simulink model "Trim"  (R2022b)
settings: Solver=ode4  StartTime=0.0  StopTime=30  FixedStep=0.01  RelTol=1e-3
undefined symbols (not defined in the file): Data, IC, Sim, v0_BE_B
libraries: simulink_extras x2, sharedutil x2
settings Model: PauseTimes=399.98  PacingRate=1000  Creator=Thoma  LastModifiedBy=muel_td
settings DataIOCC: ExternalInput=getinputstruct(report2)  InitialState=getstatestruct(report2)
settings OptimizationCC: ReuseModelBlockBuffer=on
settings DebuggingCC: AlgebraicLoopMsg=none  InitInArrayFormatMsg=none
settings RTWCC: GPUComputeCapability=5.0

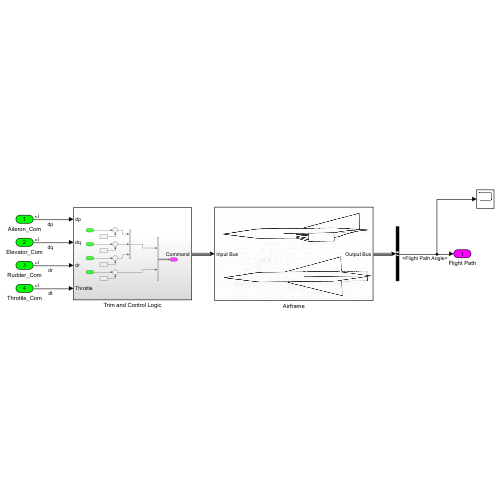
[thumbnail: Simulink's stored preview of the top-level diagram]
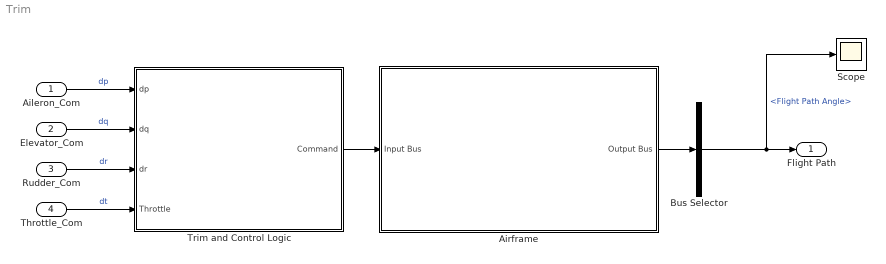
== system Trim ==
  Aileron_Com : Inport  OutDataTypeStr=double
  Elevator_Com : Inport  Port=2  OutDataTypeStr=double
  Rudder_Com : Inport  Port=3  OutDataTypeStr=double
  Throttle_Com : Inport  Port=4
  Airframe : Subsystem
      mask Display: image('GHAME.png'); % Use "Edit Image" on toolstrip to change.
  Bus Selector : BusSelector  OutputSignals=Flight Path Angle
  Scope : Scope
  Trim and Control Logic : Subsystem
  Flight Path : Outport
  wires:
  Airframe/1(Output Bus) -> Bus Selector/1
  Bus Selector/1 -> Scope/1, Flight Path/1  "<Flight Path Angle>"
  Aileron_Com/1 -> Trim and Control Logic/1(dp)  "dp"
  Elevator_Com/1 -> Trim and Control Logic/2(dq)  "dq"
  Rudder_Com/1 -> Trim and Control Logic/3(dr)  "dr"
  Throttle_Com/1 -> Trim and Control Logic/4(Throttle)  "dt"
  Trim and Control Logic/1(Command) -> Airframe/1(Input Bus)

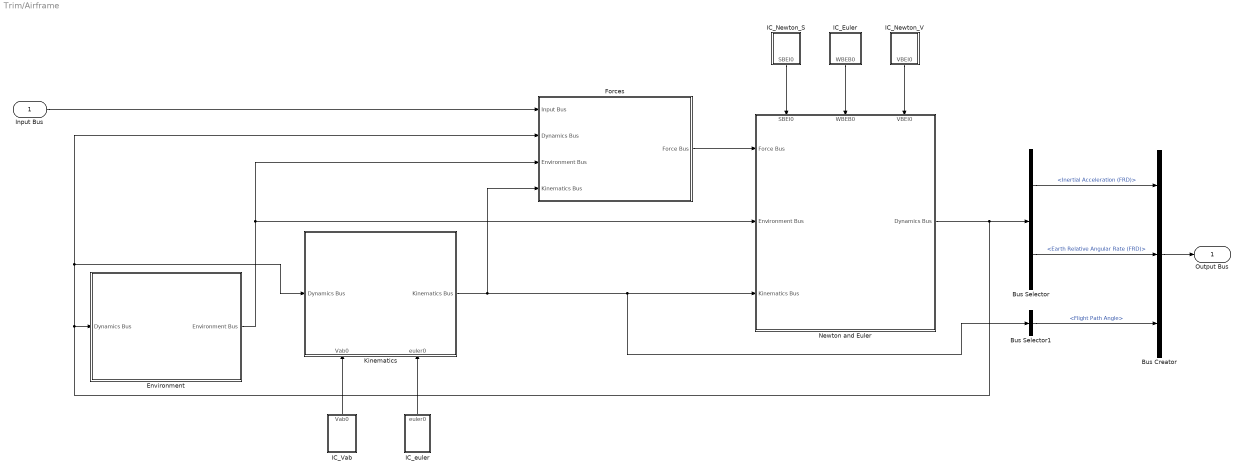
== system Trim/Airframe ==
  Input Bus : Inport
  Bus Creator : BusCreator  Inputs=3
  Bus Selector : BusSelector  OutputSignals=Inertial Acceleration (FRD),Earth Relative Angular Rate (FRD)
  Bus Selector1 : BusSelector  OutputSignals=Flight Path Angle
  Environment : Subsystem
  Forces : Subsystem
  IC_Euler : Subsystem
  IC_Newton_S : Subsystem
  IC_Newton_V : Subsystem
  IC_Vab : Subsystem
  IC_euler : Subsystem
  Kinematics : Subsystem
      settings: PortSchema="{\"entries\":[{\"content\":{\"sides\":[{\"content\":{\"connectorIds\":[\"In1\"]},\"type\":\"ConnectorPlacement.EquallySpacedRectSide\",\"uuid\":\"165cd628-1618-4ee0-958f-c15c2fb528e8\"},{\"content\":{\"connectorIds\":[\"Out1\"],\"side\":\"RIGHT\"},\"type\":\"ConnectorPlacement.EquallySpacedRectSide\",\"uuid\":\"946488ef-ac28-4d5b-ba51-e112409765b1\"},{\"content\":{\"connectorIds\":[],\"side\":\"TOP\"},\"type\":\"ConnectorPlacement.EquallySpacedRectSide\",\"uuid\":\"119c1b56-3e48-4508-9afd-e07e28cbf837\"},{\"content\":{\"connectorIds\":[\"In2\",\"In3\"],\"side\":\"BOTTOM\"},\"type\":\"ConnectorPlacement.EquallySpacedRectSide\",\"uuid\":\"d60bed97-cd35-4219-85e4-6b5accaebd4d\"}]},\"type\":\"ConnectorPlacement.EquallySpacedConnector\",\"uuid\":\"f554c72c-6bea-4d8c-bbaa-1d03e69e35ab\"}],\"packageUris\":[\"http://schema.mathworks.com/mf0/Connector/R2020b\"],\"version\":\"1.0\"}"
  Newton and Euler : Subsystem
      settings: PortSchema="{\"entries\":[{\"content\":{\"sides\":[{\"content\":{\"connectorIds\":[\"In1\",\"In2\",\"In3\"]},\"type\":\"ConnectorPlacement.EquallySpacedRectSide\",\"uuid\":\"2ee03a1f-357d-4786-8b32-c5c02601a636\"},{\"content\":{\"connectorIds\":[\"Out1\"],\"side\":\"RIGHT\"},\"type\":\"ConnectorPlacement.EquallySpacedRectSide\",\"uuid\":\"c5e575c4-9295-4acb-b0b8-b029d28de022\"},{\"content\":{\"connectorIds\":[\"In4\",\"In5\",\"In6\"],\"side\":\"TOP\"},\"type\":\"ConnectorPlacement.EquallySpacedRectSide\",\"uuid\":\"0c94ab65-bccb-43d1-9b54-9d35a0cc0e07\"}]},\"type\":\"ConnectorPlacement.EquallySpacedConnector\",\"uuid\":\"e611a102-f7b3-4598-9b4e-dc828ce04541\"}],\"packageUris\":[\"http://schema.mathworks.com/mf0/Connector/R2020b\"],\"version\":\"1.0\"}"
  Output Bus : Outport
  wires:
  Newton and Euler/1(Dynamics Bus) -> Environment/1(Dynamics Bus), Forces/2(Dynamics Bus), Kinematics/1(Dynamics Bus), Bus Selector/1
  IC_Newton_V/1(VBEI0) -> Newton and Euler/6(VBEI0)
  IC_Vab/1(Vab0) -> Kinematics/2(Vab0)
  IC_Euler/1(WBEB0) -> Newton and Euler/5(WBEB0)
  IC_Newton_S/1(SBEI0) -> Newton and Euler/4(SBEI0)
  Kinematics/1(Kinematics Bus) -> Forces/4(Kinematics Bus), Newton and Euler/3(Kinematics Bus), Bus Selector1/1
  IC_euler/1(euler0) -> Kinematics/3(euler0)
  Environment/1(Environment Bus) -> Forces/3(Environment Bus), Newton and Euler/2(Environment Bus)
  Forces/1(Force Bus) -> Newton and Euler/1(Force Bus)
  Input Bus/1 -> Forces/1(Input Bus)
  Bus Creator/1 -> Output Bus/1
  Bus Selector1/1 -> Bus Creator/3  "<Flight Path Angle>"
  Bus Selector/2 -> Bus Creator/2  "<Earth Relative Angular Rate (FRD)>"
  Bus Selector/1 -> Bus Creator/1  "<Inertial Acceleration (FRD)>"

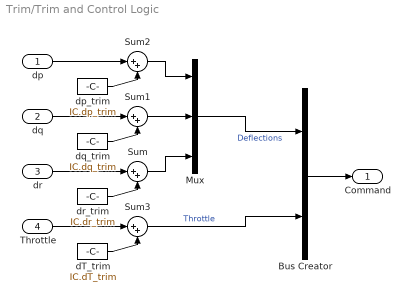
== system Trim/Trim and Control Logic ==
  dp : Inport
  dq : Inport  Port=2
  dr : Inport  Port=3
  Throttle : Inport  Port=4
  Bus Creator : BusCreator  Inputs=2
  Mux : Mux  Inputs=3
  Sum{,1..3} (4 alike) : Sum  Inputs=|++
  dT_trim : Constant  Value=IC.dT_trim
  dp_trim : Constant  Value=IC.dp_trim
  dq_trim : Constant  Value=IC.dq_trim
  dr_trim : Constant  Value=IC.dr_trim
  Command : Outport
  wires:
  dr_trim/1 -> Sum/2
  Mux/1 -> Bus Creator/1  "Deflections"
  dq_trim/1 -> Sum1/2
  dp_trim/1 -> Sum2/2
  Sum/1 -> Mux/3
  Sum2/1 -> Mux/1
  Sum1/1 -> Mux/2
  dT_trim/1 -> Sum3/2
  Sum3/1 -> Bus Creator/2  "Throttle"
  Bus Creator/1 -> Command/1
  Throttle/1 -> Sum3/1
  dr/1 -> Sum/1
  dq/1 -> Sum1/1
  dp/1 -> Sum2/1

== system Trim/Airframe/Environment ==
  Dynamics Bus : Inport
  Bus Creator : BusCreator  Inputs=5
  Bus Selector : BusSelector  OutputSignals=Geogrpahic Velocity [NED],Geodetic Altitude,Inertial Position
  ENVIRONMENT : Subsystem
      settings: PortSchema="{\"entries\":[{\"content\":{\"sides\":[{\"content\":{\"connectorIds\":[\"Out1\",\"Out2\",\"Out3\",\"Out4\",\"Out5\"]},\"type\":\"ConnectorPlacement.EquallySpacedRectSide\",\"uuid\":\"4e949b4f-5045-4889-a6e0-8d0e34c9027a\"},{\"content\":{\"connectorIds\":[\"In1\",\"In2\",\"In3\"],\"side\":\"RIGHT\"},\"type\":\"ConnectorPlacement.EquallySpacedRectSide\",\"uuid\":\"f7e1e33b-2909-4c8f-9e0b-a9d722038330\"},{\"content\":{\"connectorIds\":[],\"side\":\"TOP\"},\"type\":\"ConnectorPlacement.EquallySpacedRectSide\",\"uuid\":\"633af8e4-de1f-4d47-a61a-f33b7deb10d1\"},{\"content\":{\"connectorIds\":[],\"side\":\"BOTTOM\"},\"type\":\"ConnectorPlacement.EquallySpacedRectSide\",\"uuid\":\"a644231a-8e0c-4950-8909-9c86a5c5b308\"}]},\"type\":\"ConnectorPlacement.EquallySpacedConnector\",\"uuid\":\"4b25b4df-d0ad-4adb-940b-ab37aba9a5ef\"}],\"packageUris\":[\"http://schema.mathworks.com/mf0/Connector/R2020b\"],\"version\":\"1.0\"}"
  Environment Bus : Outport
  wires:
  ENVIRONMENT/2(rho) -> Bus Creator/2  "Air Density"
  ENVIRONMENT/1(GRAVG) -> Bus Creator/1  "Gravitation (NED)"
  ENVIRONMENT/3(pdynmc) -> Bus Creator/3  "Dynamic Pressure"
  ENVIRONMENT/5(dvba) -> Bus Creator/5  "True Airspeed"
  ENVIRONMENT/4(vmach) -> Bus Creator/4  "Mach Number"
  Bus Creator/1 -> Environment Bus/1
  Dynamics Bus/1 -> Bus Selector/1
  Bus Selector/1 -> ENVIRONMENT/1(VBED)  "<Geogrpahic Velocity [NED]>"
  Bus Selector/3 -> ENVIRONMENT/3(SBII)  "<Inertial Position>"
  Bus Selector/2 -> ENVIRONMENT/2(alt)  "<Geodetic Altitude>"

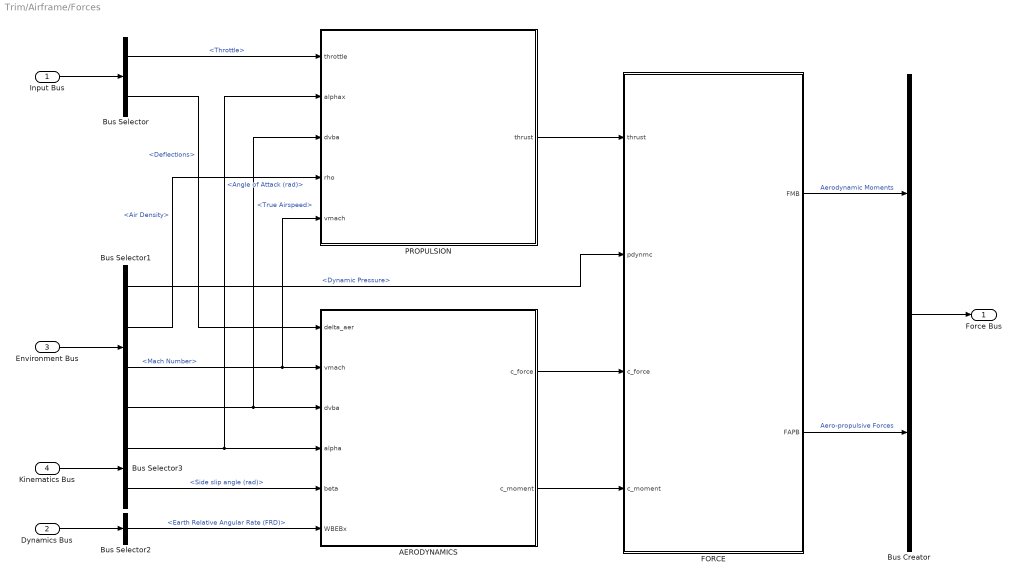
== system Trim/Airframe/Forces ==
  Input Bus : Inport
  Dynamics Bus : Inport  Port=2
  Environment Bus : Inport  Port=3
  Kinematics Bus : Inport  Port=4
  AERODYNAMICS : Subsystem
  Bus Creator : BusCreator  Inputs=2
  Bus Selector : BusSelector  OutputSignals=Throttle,Deflections
  Bus Selector1 : BusSelector  OutputSignals=Dynamic Pressure,Air Density,Mach Number,True Airspeed
  Bus Selector2 : BusSelector  OutputSignals=Earth Relative Angular Rate (FRD)
  Bus Selector3 : BusSelector  OutputSignals=Angle of Attack (rad),Side slip angle (rad)
  FORCE : Subsystem
  PROPULSION : Subsystem
  Force Bus : Outport
  wires:
  Input Bus/1 -> Bus Selector/1
  Environment Bus/1 -> Bus Selector1/1
  Bus Selector/1 -> PROPULSION/1(throttle)  "<Throttle>"
  PROPULSION/1(thrust) -> FORCE/1(thrust)
  AERODYNAMICS/1(c_force) -> FORCE/3(c_force)
  AERODYNAMICS/2(c_moment) -> FORCE/4(c_moment)
  Bus Selector1/3 -> PROPULSION/5(vmach), AERODYNAMICS/2(vmach)  "<Mach Number>"
  Bus Selector1/4 -> PROPULSION/3(dvba), AERODYNAMICS/3(dvba)  "<True Airspeed>"
  Bus Selector1/2 -> PROPULSION/4(rho)  "<Air Density>"
  Dynamics Bus/1 -> Bus Selector2/1
  Bus Selector2/1 -> AERODYNAMICS/6(WBEBx)  "<Earth Relative Angular Rate (FRD)>"
  Kinematics Bus/1 -> Bus Selector3/1
  Bus Selector3/1 -> AERODYNAMICS/4(alpha), PROPULSION/2(alphax)  "<Angle of Attack (rad)>"
  Bus Selector3/2 -> AERODYNAMICS/5(beta)  "<Side slip angle (rad)>"
  FORCE/1(FMB) -> Bus Creator/1  "Aerodynamic Moments"
  FORCE/2(FAPB) -> Bus Creator/2  "Aero-propulsive Forces"
  Bus Creator/1 -> Force Bus/1
  Bus Selector/2 -> AERODYNAMICS/1(delta_aer)  "<Deflections>"
  Bus Selector1/1 -> FORCE/2(pdynmc)  "<Dynamic Pressure>"

== system Trim/Airframe/IC_Euler ==
  Constant : Constant  Value=IC.WBIB  SampleTime=Sim.sample_time
  WBEB0 : Outport
  wires:
  Constant/1 -> WBEB0/1

== system Trim/Airframe/IC_Newton_S ==
  Constant : Constant  Value=IC.SBII  SampleTime=Sim.sample_time
  SBEI0 : Outport
  wires:
  Constant/1 -> SBEI0/1

== system Trim/Airframe/IC_Newton_V ==
  Constant : Constant  Value=IC.VBII  SampleTime=Sim.sample_time
  VBEI0 : Outport
  wires:
  Constant/1 -> VBEI0/1

== system Trim/Airframe/IC_Vab ==
  Constant : Constant  Value=[IC.dvba; IC.alpha; 0]  VectorParams1D=off  SampleTime=Sim.sample_time
  Vab0 : Outport
  wires:
  Constant/1 -> Vab0/1

== system Trim/Airframe/IC_euler ==
  Constant : Constant  Value=[IC.psibd; IC.thtbd; IC.phibd]  VectorParams1D=off  SampleTime=Sim.sample_time
  euler0 : Outport
  wires:
  Constant/1 -> euler0/1

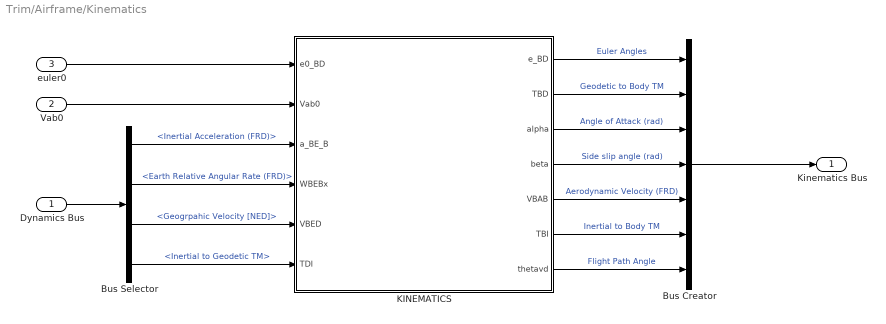
== system Trim/Airframe/Kinematics ==
  Dynamics Bus : Inport
  Vab0 : Inport  Port=2
  euler0 : Inport  Port=3
  Bus Creator : BusCreator  Inputs=7
  Bus Selector : BusSelector  OutputSignals=Inertial Acceleration (FRD),Earth Relative Angular Rate (FRD),Geogrpahic Velocity [NED],Inertial to Geodetic TM
  KINEMATICS : Subsystem
  Kinematics Bus : Outport
  wires:
  Dynamics Bus/1 -> Bus Selector/1
  Bus Selector/3 -> KINEMATICS/5(VBED)  "<Geogrpahic Velocity [NED]>"
  Bus Selector/2 -> KINEMATICS/4(WBEBx)  "<Earth Relative Angular Rate (FRD)>"
  Bus Selector/1 -> KINEMATICS/3(a_BE_B)  "<Inertial Acceleration (FRD)>"
  KINEMATICS/1(e_BD) -> Bus Creator/1  "Euler Angles"
  KINEMATICS/2(TBD) -> Bus Creator/2  "Geodetic to Body TM"
  KINEMATICS/3(alpha) -> Bus Creator/3  "Angle of Attack (rad)"
  KINEMATICS/4(beta) -> Bus Creator/4  "Side slip angle (rad)"
  KINEMATICS/5(VBAB) -> Bus Creator/5  "Aerodynamic Velocity (FRD)"
  KINEMATICS/6(TBI) -> Bus Creator/6  "Inertial to Body TM"
  Bus Creator/1 -> Kinematics Bus/1
  euler0/1 -> KINEMATICS/1(e0_BD)
  Vab0/1 -> KINEMATICS/2(Vab0)
  Bus Selector/4 -> KINEMATICS/6(TDI)  "<Inertial to Geodetic TM>"
  KINEMATICS/7(thetavd) -> Bus Creator/7  "Flight Path Angle"

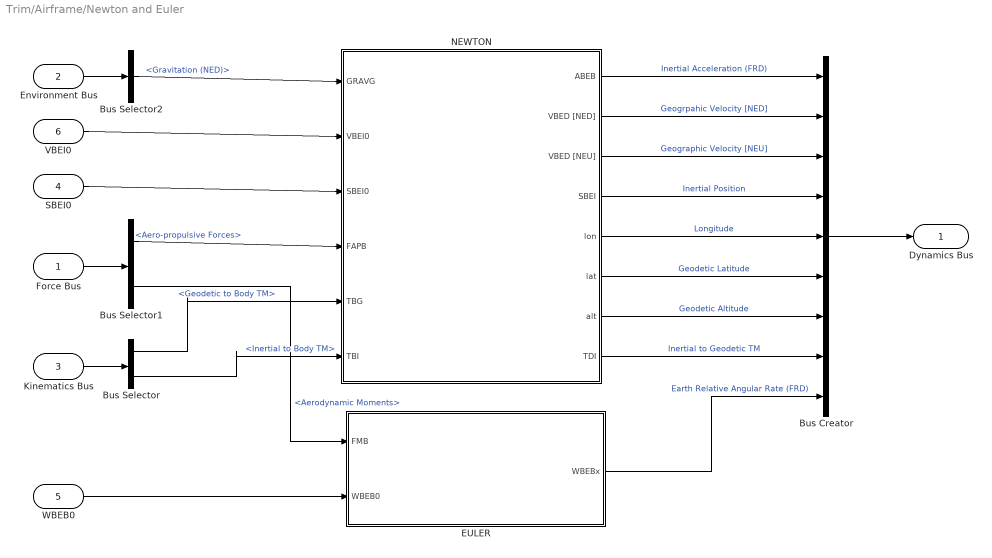
== system Trim/Airframe/Newton and Euler ==
  Force Bus : Inport
  Environment Bus : Inport  Port=2
  Kinematics Bus : Inport  Port=3
  SBEI0 : Inport  Port=4
  WBEB0 : Inport  Port=5
  VBEI0 : Inport  Port=6
  Bus Creator : BusCreator  Inputs=9
  Bus Selector : BusSelector  OutputSignals=Geodetic to Body TM,Inertial to Body TM
  Bus Selector1 : BusSelector  OutputSignals=Aero-propulsive Forces,Aerodynamic Moments
  Bus Selector2 : BusSelector  OutputSignals=Gravitation (NED)
  EULER : Subsystem
  NEWTON : Subsystem
      settings: PortSchema="{\"entries\":[{\"content\":{\"sides\":[{\"content\":{},\"type\":\"ConnectorPlacement.EquallySpacedRectSide\",\"uuid\":\"0afd3c46-ebac-4ac7-882c-33fd81ca5d64\"},{\"content\":{\"side\":\"RIGHT\"},\"type\":\"ConnectorPlacement.EquallySpacedRectSide\",\"uuid\":\"c4cd72f8-7163-4cf6-9ccc-a17ef192f179\"},{\"content\":{\"connectorIds\":[\"In1\",\"In2\",\"In3\",\"In4\",\"In5\",\"In6\"],\"side\":\"TOP\"},\"type\":\"ConnectorPlacement.EquallySpacedRectSide\",\"uuid\":\"bacc7392-75fb-4735-9a46-243c92f3a88e\"},{\"content\":{\"connectorIds\":[\"Out1\",\"Out2\",\"Out3\",\"Out4\",\"Out5\",\"Out6\",\"Out7\",\"Out8\"],\"side\":\"BOTTOM\"},\"type\":\"ConnectorPlacement.EquallySpacedRectSide\",\"uuid\":\"cef8e5ca-fd27-4ea3-ab26-80916cc697cd\"}]},\"type\":\"ConnectorPlacement.EquallySpacedConnector\",\"uuid\":\"94e5b9d6-625b-42c3-8a13-a4958692d432\"}],\"packageUris\":[\"http://schema.mathworks.com/mf0/Connector/R2020b\"],\"version\":\"1.0\"}"
  Dynamics Bus : Outport
  wires:
  WBEB0/1 -> EULER/2(WBEB0)
  Bus Selector1/2 -> EULER/1(FMB)  "<Aerodynamic Moments>"
  Bus Selector1/1 -> NEWTON/4(FAPB)  "<Aero-propulsive Forces>"
  VBEI0/1 -> NEWTON/2(VBEI0)
  SBEI0/1 -> NEWTON/3(SBEI0)
  Bus Creator/1 -> Dynamics Bus/1
  NEWTON/1(ABEB) -> Bus Creator/1  "Inertial Acceleration (FRD)"
  NEWTON/2(VBED [NED]) -> Bus Creator/2  "Geogrpahic Velocity [NED]"
  NEWTON/3(VBED [NEU]) -> Bus Creator/3  "Geographic Velocity [NEU]"
  NEWTON/4("SBEI ") -> Bus Creator/4  "Inertial Position"
  NEWTON/5(lon) -> Bus Creator/5  "Longitude"
  NEWTON/6(lat) -> Bus Creator/6  "Geodetic Latitude"
  NEWTON/7(alt) -> Bus Creator/7  "Geodetic Altitude"
  Kinematics Bus/1 -> Bus Selector/1
  Bus Selector/2 -> NEWTON/6(TBI)  "<Inertial to Body TM>"
  Force Bus/1 -> Bus Selector1/1
  Bus Selector/1 -> NEWTON/5(TBG)  "<Geodetic to Body TM>"
  Environment Bus/1 -> Bus Selector2/1
  Bus Selector2/1 -> NEWTON/1(GRAVG)  "<Gravitation (NED)>"
  NEWTON/8(TDI) -> Bus Creator/8  "Inertial to Geodetic TM"
  EULER/1(WBEBx) -> Bus Creator/9  "Earth Relative Angular Rate (FRD)"

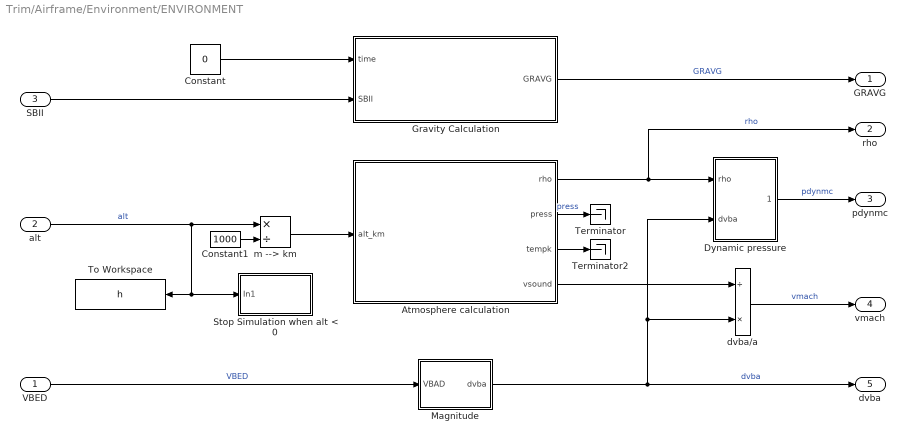
== system Trim/Airframe/Environment/ENVIRONMENT ==
  VBED : Inport
  alt : Inport  Port=2
  SBII : Inport  Port=3
  Atmosphere calculation : MATLAB Function  Priority=2  TreatAsAtomicUnit=on
  Constant : Constant  Value=0
  Constant1 : Constant  Value=1000
  Dynamic pressure : Subsystem
  Gravity Calculation : MATLAB Function  Priority=1  TreatAsAtomicUnit=on
  Magnitude : MATLAB Function  TreatAsAtomicUnit=on
  Stop Simulation when alt < 0 : Subsystem
  Terminator : Terminator
  Terminator2 : Terminator
  To Workspace : ToWorkspace  VariableName=h  SampleTime=-1
  dvba/a : Product  Inputs=/*
  m --> km : Product  Inputs=*/
  GRAVG : Outport
  rho : Outport  Port=2
  pdynmc : Outport  Port=3
  vmach : Outport  Port=4
  dvba : Outport  Port=5
  wires:
  alt/1 -> To Workspace/1, Stop Simulation when alt < 0/1(In1), m --> km/1  "alt"
  Atmosphere calculation/3(tempk) -> Terminator2/1
  Constant1/1 -> m --> km/2
  m --> km/1 -> Atmosphere calculation/1(alt_km)
  dvba/a/1 -> vmach/1  "vmach"
  Atmosphere calculation/1(rho) -> Dynamic pressure/1(rho), rho/1  "rho"
  Dynamic pressure/1(pdynmc) -> pdynmc/1  "pdynmc"
  Atmosphere calculation/4(vsound) -> dvba/a/1
  Magnitude/1(dvba) -> dvba/a/2, Dynamic pressure/2(dvba), dvba/1  "dvba"
  Constant/1 -> Gravity Calculation/1(time)
  Gravity Calculation/1(GRAVG) -> GRAVG/1  "GRAVG"
  SBII/1 -> Gravity Calculation/2(SBII)
  VBED/1 -> Magnitude/1(VBAD)  "VBED"
  Atmosphere calculation/2(press) -> Terminator/1  "press"

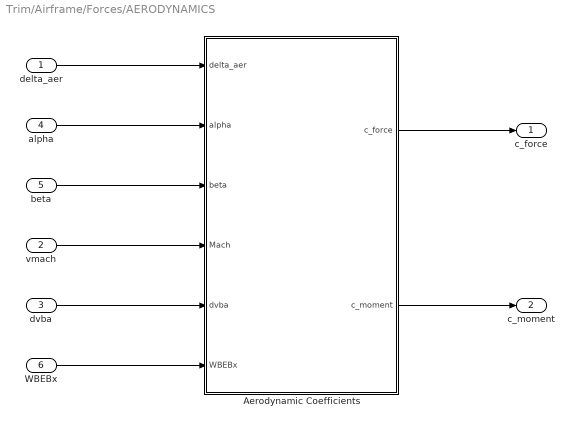
== system Trim/Airframe/Forces/AERODYNAMICS ==
  delta_aer : Inport
  vmach : Inport  Port=2
  dvba : Inport  Port=3
  alpha : Inport  Port=4
  beta : Inport  Port=5
  WBEBx : Inport  Port=6
  Aerodynamic Coefficients : MATLAB Function  TreatAsAtomicUnit=on
  c_force : Outport  PortDimensions=[3 1]
  c_moment : Outport  Port=2  PortDimensions=[3 1]
  wires:
  vmach/1 -> Aerodynamic Coefficients/4(Mach)
  dvba/1 -> Aerodynamic Coefficients/5(dvba)
  beta/1 -> Aerodynamic Coefficients/3(beta)
  alpha/1 -> Aerodynamic Coefficients/2(alpha)
  Aerodynamic Coefficients/1(c_force) -> c_force/1
  WBEBx/1 -> Aerodynamic Coefficients/6(WBEBx)
  Aerodynamic Coefficients/2(c_moment) -> c_moment/1
  delta_aer/1 -> Aerodynamic Coefficients/1(delta_aer)

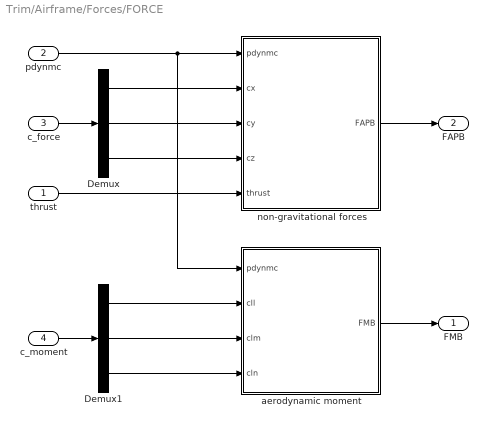
== system Trim/Airframe/Forces/FORCE ==
  thrust : Inport
  pdynmc : Inport  Port=2
  c_force : Inport  Port=3  PortDimensions=[3 1]
  c_moment : Inport  Port=4  PortDimensions=[3 1]
  Demux : Demux  Outputs=3
  Demux1 : Demux  Outputs=3
  aerodynamic moment : MATLAB Function  TreatAsAtomicUnit=on
  non-gravitational forces : MATLAB Function  TreatAsAtomicUnit=on
  FMB : Outport
  FAPB : Outport  Port=2
  wires:
  Demux/1 -> non-gravitational forces/2(cx)
  c_force/1 -> Demux/1
  Demux/3 -> non-gravitational forces/4(cz)
  non-gravitational forces/1(FAPB) -> FAPB/1
  Demux1/1 -> aerodynamic moment/2(cll)
  c_moment/1 -> Demux1/1
  Demux1/3 -> aerodynamic moment/4(cln)
  aerodynamic moment/1(FMB) -> FMB/1
  Demux/2 -> non-gravitational forces/3(cy)
  Demux1/2 -> aerodynamic moment/3(clm)
  thrust/1 -> non-gravitational forces/5(thrust)
  pdynmc/1 -> non-gravitational forces/1(pdynmc), aerodynamic moment/1(pdynmc)

== system Trim/Airframe/Forces/PROPULSION ==
  throttle : Inport
  alphax : Inport  Port=2
  dvba : Inport  Port=3
  rho : Inport  Port=4
  vmach : Inport  Port=5
  making thrust calculations : MATLAB Function  TreatAsAtomicUnit=on
  thrust : Outport
  wires:
  rho/1 -> making thrust calculations/1(rho)
  dvba/1 -> making thrust calculations/4(DVBA)
  vmach/1 -> making thrust calculations/2(Mach)
  making thrust calculations/1(Thrust) -> thrust/1  "Thrust"
  alphax/1 -> making thrust calculations/3(alphax)
  throttle/1 -> making thrust calculations/5(Throttle)

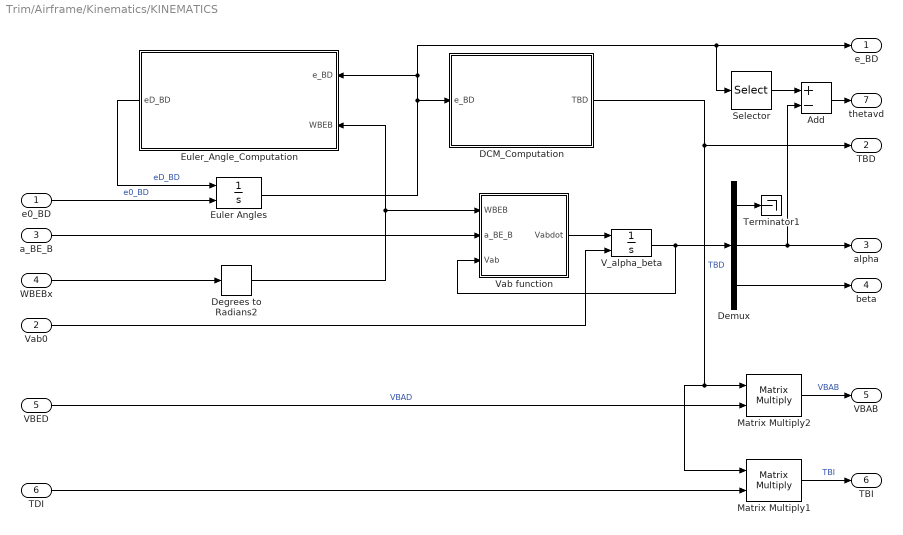
== system Trim/Airframe/Kinematics/KINEMATICS ==
  e0_BD : Inport
  Vab0 : Inport  Port=2
  a_BE_B : Inport  Port=3
  WBEBx : Inport  Port=4
  VBED : Inport  Port=5
  TDI : Inport  Port=6
  Add : Sum  Inputs=+-
  DCM_Computation : MATLAB Function  TreatAsAtomicUnit=on
  Degrees to Radians2 : simulink_extras/Transformations/Degrees to Radians
  Demux : Demux  Outputs=3
  Euler Angles : Integrator  InitialConditionSource=external
  Euler_Angle_Computation : MATLAB Function  TreatAsAtomicUnit=on
  Matrix Multiply1 : Product  Multiplication=Matrix(*)
  Matrix Multiply2 : Product  Multiplication=Matrix(*)
  Selector : Selector  InputPortWidth=3  IndexOptions=Index vector (dialog)  Indices=[2]  OutputSizes=1
  Terminator1 : Terminator
  V_alpha_beta : Integrator  InitialConditionSource=external
  Vab function : MATLAB Function  TreatAsAtomicUnit=on
  e_BD : Outport
  TBD : Outport  Port=2
  alpha : Outport  Port=3
  beta : Outport  Port=4
  VBAB : Outport  Port=5
  TBI : Outport  Port=6
  thetavd : Outport  Port=7
  wires:
  Matrix Multiply1/1 -> TBI/1  "TBI"
  VBED/1 -> Matrix Multiply2/2  "VBAD"
  WBEBx/1 -> Degrees to Radians2/1
  Euler Angles/1 -> e_BD/1, Selector/1, Euler_Angle_Computation/1(e_BD), DCM_Computation/1(e_BD)
  DCM_Computation/1(TBD) -> TBD/1, Matrix Multiply1/1, Matrix Multiply2/1  "TBD"
  e0_BD/1 -> Euler Angles/2  "e0_BD"
  Euler_Angle_Computation/1(eD_BD) -> Euler Angles/1  "eD_BD"
  Vab function/1(Vabdot) -> V_alpha_beta/1
  Vab0/1 -> V_alpha_beta/2
  V_alpha_beta/1 -> Vab function/3(Vab), Demux/1
  Demux/1 -> Terminator1/1
  Demux/3 -> beta/1
  a_BE_B/1 -> Vab function/2(a_BE_B)
  Degrees to Radians2/1 -> Vab function/1(WBEB), Euler_Angle_Computation/2(WBEB)
  Demux/2 -> alpha/1, Add/2
  Matrix Multiply2/1 -> VBAB/1  "VBAB"
  TDI/1 -> Matrix Multiply1/2
  Selector/1 -> Add/1
  Add/1 -> thetavd/1

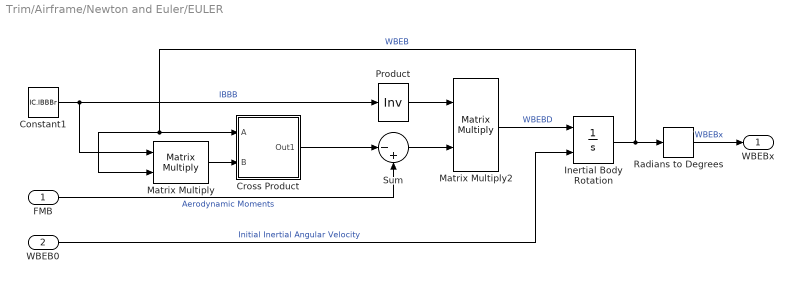
== system Trim/Airframe/Newton and Euler/EULER ==
  FMB : Inport
  WBEB0 : Inport  Port=2
  Constant1 : Constant  Value=IC.IBBBr
  Cross Product : Subsystem
  Inertial Body Rotation : Integrator  InitialConditionSource=external  InitialCondition=v0_BE_B
  Matrix Multiply : Product  Multiplication=Matrix(*)
  Matrix Multiply2 : Product  Multiplication=Matrix(*)
  Product : Product  Inputs=/  Multiplication=Matrix(*)  SaturateOnIntegerOverflow=on  OutDataTypeStr=Inherit: Same as first input
  Radians to Degrees : simulink_extras/Transformations/Radians to Degrees
  Sum : Sum  Inputs=|-+
  WBEBx : Outport
  wires:
  FMB/1 -> Sum/2  "Aerodynamic Moments"
  Matrix Multiply2/1 -> Inertial Body Rotation/1  "WBEBD"
  Constant1/1 -> Product/1, Matrix Multiply/1  "IBBB"
  Inertial Body Rotation/1 -> Radians to Degrees/1, Cross Product/1(A), Matrix Multiply/2  "WBEB"
  Product/1 -> Matrix Multiply2/1
  Matrix Multiply/1 -> Cross Product/2(B)
  Sum/1 -> Matrix Multiply2/2
  WBEB0/1 -> Inertial Body Rotation/2  "Initial Inertial Angular Velocity"
  Radians to Degrees/1 -> WBEBx/1  "WBEBx"
  Cross Product/1(Out1) -> Sum/1

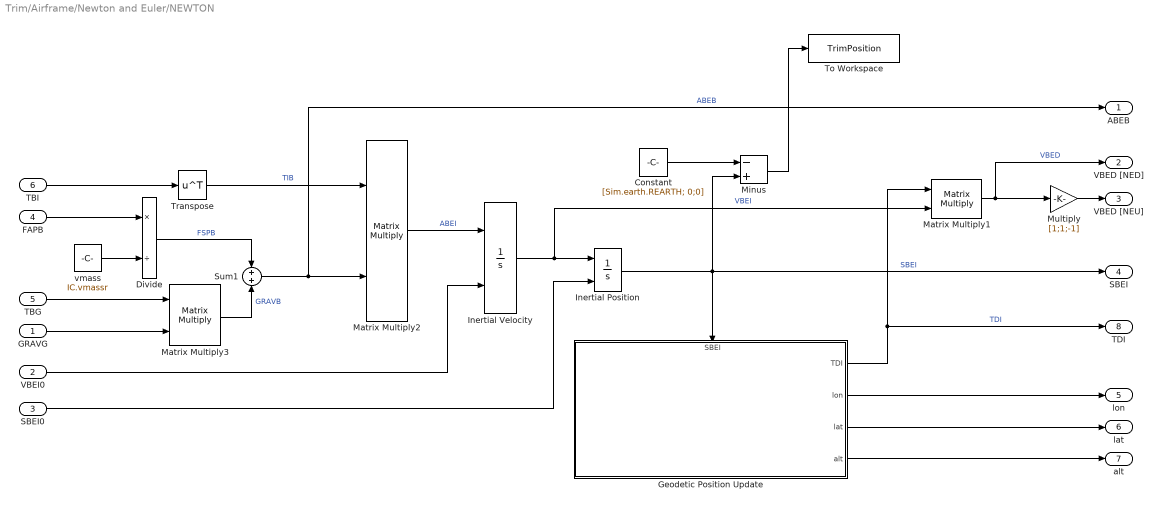
== system Trim/Airframe/Newton and Euler/NEWTON ==
  GRAVG : Inport
  VBEI0 : Inport  Port=2
  SBEI0 : Inport  Port=3
  FAPB : Inport  Port=4
  TBG : Inport  Port=5
  TBI : Inport  Port=6
  Constant : Constant  Value=[Sim.earth.REARTH; 0;0]  SampleTime=Sim.sample_time
  Divide : Product  Inputs=*/
  Geodetic Position Update : Subsystem
      settings: PortSchema="{\"entries\":[{\"content\":{\"sides\":[{\"content\":{\"connectorIds\":[\"Out1\",\"Out2\",\"Out3\",\"Out4\"]},\"type\":\"ConnectorPlacement.EquallySpacedRectSide\",\"uuid\":\"354b3e00-ca99-4fc7-9992-405a02a040f5\"},{\"content\":{\"side\":\"RIGHT\"},\"type\":\"ConnectorPlacement.EquallySpacedRectSide\",\"uuid\":\"8f955005-4883-4776-afdd-d407599bb461\"},{\"content\":{\"connectorIds\":[\"In1\"],\"side\":\"TOP\"},\"type\":\"ConnectorPlacement.EquallySpacedRectSide\",\"uuid\":\"76f4e1b5-15b6-4413-a3b6-5a25f7ad2dec\"}]},\"type\":\"ConnectorPlacement.EquallySpacedConnector\",\"uuid\":\"e91e95e0-c229-454d-8b62-a3f0d70a30c5\"}],\"packageUris\":[\"http://schema.mathworks.com/mf0/Connector/R2020b\"],\"version\":\"1.0\"}"
  Inertial Position : Integrator  InitialConditionSource=external
  Inertial Velocity : Integrator  InitialConditionSource=external  InitialCondition=v0_BE_B
  Matrix Multiply1 : Product  Multiplication=Matrix(*)
  Matrix Multiply2 : Product  Multiplication=Matrix(*)
  Matrix Multiply3 : Product  Multiplication=Matrix(*)
  Minus : Sum  Inputs=-+
  Multiply : Gain  Gain=[1;1;-1]
  Sum1 : Sum
  To Workspace : ToWorkspace  VariableName=TrimPosition  SaveFormat=Timeseries  SampleTime=-1
  Transpose : Math  Operator=transpose
  vmass : Constant  Value=IC.vmassr
  ABEB : Outport
  VBED [NED] : Outport  Port=2
  VBED [NEU] : Outport  Port=3
  "SBEI " : Outport  Port=4
  lon : Outport  Port=5
  lat : Outport  Port=6
  alt : Outport  Port=7
  TDI : Outport  Port=8
  wires:
  TBG/1 -> Matrix Multiply3/1
  GRAVG/1 -> Matrix Multiply3/2
  Divide/1 -> Sum1/1  "FSPB"
  Sum1/1 -> ABEB/1, Matrix Multiply2/2  "ABEB"
  vmass/1 -> Divide/2
  Matrix Multiply1/1 -> Multiply/1, VBED [NED]/1  "VBED"
  FAPB/1 -> Divide/1
  Matrix Multiply3/1 -> Sum1/2  "GRAVB"
  Multiply/1 -> VBED [NEU]/1
  VBEI0/1 -> Inertial Velocity/2
  Inertial Velocity/1 -> Matrix Multiply1/2, Inertial Position/1  "VBEI"
  SBEI0/1 -> Inertial Position/2
  Inertial Position/1 -> "SBEI "/1, Minus/2, Geodetic Position Update/1(SBEI)  "SBEI"
  Matrix Multiply2/1 -> Inertial Velocity/1  "ABEI"
  TBI/1 -> Transpose/1
  Transpose/1 -> Matrix Multiply2/1  "TIB"
  Geodetic Position Update/1(TDI) -> TDI/1, Matrix Multiply1/1  "TDI"
  Geodetic Position Update/4(alt) -> alt/1
  Geodetic Position Update/3(lat) -> lat/1
  Geodetic Position Update/2(lon) -> lon/1
  Constant/1 -> Minus/1
  Minus/1 -> To Workspace/1

== system Trim/Airframe/Environment/ENVIRONMENT/Dynamic pressure ==
  rho : Inport
  dvba : Inport  Port=2
  Gain : Gain  Gain=0.5
  Product : Product
  Square : Math  Operator=square
  pdynmc : Outport
  wires:
  Gain/1 -> pdynmc/1
  Product/1 -> Gain/1
  rho/1 -> Product/2
  dvba/1 -> Square/1
  Square/1 -> Product/1

== system Trim/Airframe/Environment/ENVIRONMENT/Stop Simulation when alt < 0 ==
  In1 : Inport
  If : If  IfExpression=u1 <= 25  ShowElse=off
  Stop Simulationalt<0 : Subsystem  TreatAsAtomicUnit=on
  wires:
  If/1 -> Stop Simulationalt<0/Action
  In1/1 -> If/1

== system Trim/Airframe/Newton and Euler/EULER/Cross Product ==
  A : Inport
  B : Inport  Port=2
  Subsystem : sharedutil/3x3 Cross Product/Subsystem  SystemSampleTime=-1  VariantActivationTime=update diagram  Latency=0  AutoFrameSizeCalculation=off
  Subsystem1 : sharedutil/3x3 Cross Product/Subsystem1  SystemSampleTime=-1  VariantActivationTime=update diagram  Latency=0  AutoFrameSizeCalculation=off
  Sum : Sum  Inputs=+|-  InputSameDT=on  SaturateOnIntegerOverflow=on  OutDataTypeStr=Inherit: Same as first input
  Out1 : Outport
  wires:
  Subsystem/1 -> Sum/1
  B/1 -> Subsystem/2, Subsystem1/2
  A/1 -> Subsystem1/1, Subsystem/1
  Subsystem1/1 -> Sum/2
  Sum/1 -> Out1/1

== system Trim/Airframe/Newton and Euler/NEWTON/Geodetic Position Update ==
  SBEI : Inport
  Find Geodetic Position : MATLAB Function  TreatAsAtomicUnit=on
  Inertial to Geodetic : MATLAB Function  TreatAsAtomicUnit=on
  TDI : Outport
  lon : Outport  Port=2
  lat : Outport  Port=3
  alt : Outport  Port=4
  wires:
  SBEI/1 -> Find Geodetic Position/1(SBII)
  Find Geodetic Position/1(lon) -> Inertial to Geodetic/1("lon ")
  Find Geodetic Position/2(lat) -> Inertial to Geodetic/2("lat ")
  Find Geodetic Position/3(alt) -> Inertial to Geodetic/3("alt ")
  Inertial to Geodetic/1(TDI) -> TDI/1  "TDI"
  Inertial to Geodetic/4(alt) -> alt/1
  Inertial to Geodetic/3(lon) -> lon/1
  Inertial to Geodetic/2(lat) -> lat/1

== system Trim/Airframe/Environment/ENVIRONMENT/Stop Simulation when alt < 0/Stop Simulationalt<0 ==
  Action Port : ActionPort  ActionPortLabel=if(u1 <= 25)
  Constant2 : Constant
  Stop Simulation : Stop
  wires:
  Constant2/1 -> Stop Simulation/1

== matlab function Trim/Airframe/Environment/ENVIRONMENT/Gravity Calculation ==
  data: time input; SBII input; GRAVG output; Sim parameter
function GRAVG  = cad_grav84(time, SBII, Sim)
  
    SMAJOR_AXIS = Sim.earth.SMAJOR_AXIS;
    C20         = Sim.earth.C20 ;
    REARTH      = Sim.earth.REARTH;
    GW_CLONG    = Sim.earth.GW_CLONG;
    GM          = Sim.earth.GM ;
    WEII3       = Sim.earth.WEII3;
    % Initialize output
    GRAVG = zeros(3,1);

    % Compute geocentric coordinates
    [lonc, latc, altc] = cad_geoc_in(SBII, time, REARTH, WEII3, GW_CLONG);

    % Compute the gravitational acceleration
    dbi = norm(SBII); % Magnitude of position vector
    dum1 = GM / (dbi^2);
    dum2 = 3 * sqrt(5);
    dum3 = (SMAJOR_AXIS / dbi)^2;

    gravg1 = -dum1 * dum2 * C20 * dum3 * sin(latc) * cos(latc);
    gravg2 = 0;
    gravg3 = dum1 * (1 + dum2 / 2 * C20 * dum3 * (3 * sin(latc)^2 - 1));

    % Assign values
    GRAVG(1) = gravg1;
    GRAVG(2) = gravg2;
    GRAVG(3) = gravg3;
end

function [lonc, latc, altc] = cad_geoc_in(SBII, time, REARTH, WEII3, GW_CLONG)

    % Extract position components
    sbii1 = SBII(1);
    sbii2 = SBII(2);
    sbii3 = SBII(3);

    % Compute geodetic latitude
    dbi = norm(SBII);
    latc = asin(sbii3 / dbi);

    % Compute altitude
    altc = dbi - REARTH;

    % Compute longitude
    dum4 = asin(sbii2 / sqrt(sbii1^2 + sbii2^2));

    % Resolving multi-valued arcsin function
    if sbii1 >= 0 && sbii2 >= 0
        lon_cel = dum4; % Quadrant I
    elseif sbii1 < 0 && sbii2 >= 0
        lon_cel = pi - dum4; % Quadrant II
    elseif sbii1 < 0 && sbii2 < 0
        lon_cel = pi - dum4; % Quadrant III
    else
        lon_cel = 2 * pi + dum4; % Quadrant IV
    end

    lonc = lon_cel - WEII3 * time - GW_CLONG;

    % Adjust longitude to be in the range (-pi, pi)
    if lonc > pi
        lonc = -(2 * pi - lonc);
    end
end

== matlab function Trim/Airframe/Kinematics/KINEMATICS/DCM_Computation ==
  data: TBD output; e_BD input
function TBD  = DCM_Computation(e_BD)

%% Inputs

% Euler angles (BVR)
phi_B   = e_BD(1,1);
theta_B = e_BD(2,1);
psi_B   = e_BD(3,1);

%% DCM computation

% Euler angles (BVR)
phi_B   = phi_B - 2*pi*floor((phi_B+pi)/(2*pi));    % -pi   <= phi   <= +pi

% DCM matrix (BVR)
TBD = [+cos(psi_B)*cos(theta_B)                                  +sin(psi_B)*cos(theta_B)                                  -sin(theta_B);...
        +cos(psi_B)*sin(theta_B)*sin(phi_B)-sin(psi_B)*cos(phi_B) +sin(psi_B)*sin(theta_B)*sin(phi_B)+cos(psi_B)*cos(phi_B) +cos(theta_B)*sin(phi_B);...
        +cos(psi_B)*sin(theta_B)*cos(phi_B)+sin(psi_B)*sin(phi_B) +sin(psi_B)*sin(theta_B)*cos(phi_B)-cos(psi_B)*sin(phi_B) +cos(theta_B)*cos(phi_B)];

% Orthogonality
TBD = TBD + (1/2)*(eye(3)-TBD*TBD')*TBD;

== matlab function Trim/Airframe/Kinematics/KINEMATICS/Euler_Angle_Computation ==
  data: e_BD input; WBEB input; eD_BD output
function eD_BD = Euler_Angle_Computation(e_BD, WBEB)

%% Inputs

% Euler angles (BVR)
phi_B   = e_BD(1,1);
theta_B = e_BD(2,1);
psi_B   = e_BD(3,1); 

%% Auxiliary variables

% AK matrix
T_edotomega = [1 +sin(phi_B)*tan(theta_B) +cos(phi_B)*tan(theta_B);...
               0 +cos(phi_B)              -sin(phi_B);...
               0 +sin(phi_B)*sec(theta_B) +cos(phi_B)*sec(theta_B)];

%% Euler angle computation

% Euler angle rate (BVR)     
eD_BD = T_edotomega*WBEB;   

%% Outputs

== matlab function Trim/Airframe/Kinematics/KINEMATICS/Vab function ==
  data: WBEB input; a_BE_B input; Vab input; Vabdot output
function Vabdot = fcn(WBEB, a_BE_B, Vab)

V     = Vab(1);
alpha = Vab(2);
beta  = Vab(3);

p = WBEB(1);
q = WBEB(2);
r = WBEB(3);

%% Auxiliary variables

u = V*cos(alpha)*cos(beta);
v = V*sin(beta);
w = V*sin(alpha)*cos(beta);

%% Translational Dynamics (TD)

% Compute matrices
T1 = [0;...
      q - (p*cos(alpha) + r*sin(alpha))*tan(beta);...
      p*sin(alpha) - r*cos(alpha)];

T2 = [V*cos(alpha)*cos(beta) V*sin(beta) V*sin(alpha)*cos(beta);...
       -sin(alpha)/cos(beta)  0            cos(alpha)/cos(beta);...
       -cos(alpha)*sin(beta)  cos(beta)   -sin(alpha)*sin(beta)];

% Compute dynamics
Vabdot = T1 + (1/V)*T2*a_BE_B;

== matlab function Trim/Airframe/Forces/AERODYNAMICS/Aerodynamic Coefficients ==
  data: delta_aer input; c_force output double size=[3 1]; alpha input; beta input; Mach input; dvba input; WBEBx input; c_moment output double size=[3 1]; Data parameter; Sim parameter
function [c_force, c_moment] = AeroCoefficients_Computation(delta_aer, alpha, beta, Mach, dvba, WBEBx, Data, Sim)

% Conversions
RAD = Sim.constants.RAD;
DEG = Sim.constants.DEG;

refb = Sim.vehicle.geometry.refb; 
refc = Sim.vehicle.geometry.refc;

delax = delta_aer(1)*DEG;
delex = delta_aer(2)*DEG;
delrx = delta_aer(3)*DEG;

ppx = WBEBx(1);
qqx = WBEBx(2);
rrx = WBEBx(3);

alphax = alpha*DEG;
betax  = beta *DEG;

AeroCoefficients = Data.AeroCoefficients;

% Coefficients
CL1_tab     =   AeroCoefficients.CL1_tab;
Cm1_tab     =   AeroCoefficients.Cm1_tab;
CD1_tab     =   AeroCoefficients.CD1_tab;

% Breakpoints
alpha_vec = -3:3:21;  % length 9
mach_vec = [0.4 0.6 0.8 0.9 0.95 1.05 1.2 1.5 2.0 3.0 6.0 12.0 24.0];  % length 13

% Helper interpolation function
interp_coeff = @(table) interp2(mach_vec, alpha_vec, table, Mach, alphax, 'linear');

% Indexed model
Cm1 = interp2(mach_vec, alpha_vec, Cm1_tab,  Mach, alphax, 'linear');
CL1 = interp2(mach_vec, alpha_vec, CL1_tab,  Mach, alphax, 'linear');
CD1 = interp2(mach_vec, alpha_vec, CD1_tab,  Mach, alphax, 'linear');

% Drag
cd0 = interp_coeff(AeroCoefficients.CD0_tab);
cda = interp_coeff(AeroCoefficients.CDA_tab);
cd  = CD1;

% Lift
cl0  = interp_coeff(AeroCoefficients.CL0_tab);
cla  = interp_coeff(AeroCoefficients.CLA_tab);
clde = interp_coeff(AeroCoefficients.CLDE_tab);
cl   = CL1 + clde * delex;

% Side force
cyb  = interp_coeff(AeroCoefficients.CYB_tab);
cyda = interp_coeff(AeroCoefficients.CYDA_tab);
cydr = interp_coeff(AeroCoefficients.CYDR_tab);
cy   = cyb * betax + cyda * delax + cydr * delrx;

% Rolling moment
cllb  = interp_coeff(AeroCoefficients.CLLB_tab);
cllda = interp_coeff(AeroCoefficients.CLLDA_tab);
clldr = interp_coeff(AeroCoefficients.CLLDR_tab);
cllp  = interp_coeff(AeroCoefficients.CLLP_tab);
cllr  = interp_coeff(AeroCoefficients.CLLR_tab);
cll   = cllb * betax + cllda * delax + clldr * delrx + cllp * ppx * RAD * refb / (2 * dvba) + cllr * rrx * RAD * refb / (2 * dvba);

% Pitching moment
cm0   = interp_coeff(AeroCoefficients.CM0_tab);
cma   = interp_coeff(AeroCoefficients.CMA_tab);
cmde  = interp_coeff(AeroCoefficients.CMDE_tab);
cmq   = interp_coeff(AeroCoefficients.CMQ_tab);
clm   = Cm1 + cmde * delex + cmq * qqx * RAD * refc / (2 * dvba);

% Yawing moment
clnb  = interp_coeff(AeroCoefficients.CNB_tab);
clnda = interp_coeff(AeroCoefficients.CNDA_tab);
clndr = interp_coeff(AeroCoefficients.CNDR_tab);
clnp  = interp_coeff(AeroCoefficients.CNP_tab);
clnr  = interp_coeff(AeroCoefficients.CNR_tab);
cln   = clnb * betax + clnda * delax + clndr * delrx + clnp * ppx * RAD * refb / (2 * dvba) + clnr * rrx * RAD * refb / (2 * dvba);

%Force coefficients in body coord
cosa = cos(alphax*RAD);
sina = sin(alphax*RAD);

cx = -cd * cosa + cl * sina;
cz = -cd * sina - cl * cosa;

c_force  = [cx; cy; cz];
c_moment = [cll; clm; cln];

end

== matlab function Trim/Airframe/Forces/FORCE/aerodynamic moment ==
  data: pdynmc input; FMB output; cll input; clm input; cln input; Sim parameter
function FMB = computeMoment(pdynmc, cll, clm, cln, Sim)
    % Compute aerodynamic moment
    % Inputs:
    %   pdynmc  - Dynamic pressure
    %   cll, clm, cln - Aerodynamic moment coefficients
    %
    % Output:
    %   FMB - 3x1 vector of aerodynamic moments in the body frame

    refa = Sim.vehicle.geometry.refa;
    refb = Sim.vehicle.geometry.refb; 
    refc = Sim.vehicle.geometry.refc;
    
    FMB = [pdynmc * refa * refb * cll; 
           pdynmc * refa * refc * clm; 
           pdynmc * refa * refb * cln];
end

== matlab function Trim/Airframe/Forces/FORCE/non-gravitational forces ==
  data: pdynmc input; FAPB output size=[3 1]; cx input; cy input; cz input; thrust input; Sim parameter
function FAPB = computeForces(pdynmc, cx, cy, cz, thrust, Sim)
    % Compute total non-gravitational forces
    % Inputs:
    %   pdynmc  - Dynamic pressure
    %   cx, cy, cz - Aerodynamic force coefficients
    %   thrust  - Thrust force along x-direction
    %
    % Output:
    %   FAPB - 3x1 vector of forces in the body frame

    refa = Sim.vehicle.geometry.refa;
    
    FAPB = [pdynmc * refa * cx + thrust; 
            pdynmc * refa * cy ; 
            pdynmc * refa * cz];
end

== matlab function Trim/Airframe/Forces/PROPULSION/making thrust calculations ==
  data: rho input; Mach input; alphax input; DVBA input; Thrust output; Data parameter; Throttle input; Sim parameter
function Thrust = thrust(rho, Mach, alphax, DVBA, Data, Throttle, Sim)
% thrust
% -------------------------------------------------------------------------
% Computes the engine thrust, fuel mass depletion rate, and propulsive
% force coefficient for the vehicle. Thrust is modeled as a function of
% Mach number, throttle setting, angle of attack, and atmospheric density.
%
% INPUTS:
%   rho          - Atmospheric density [kg/m^3]
%   Mach         - Mach number [-]
%   alphax       - Angle of attack [rad]
%   DVBA         - True airspeed (speed of vehicle wrt air) [m/s]
%   Data         - Struct with engine coefficient tables:
%                    Data.Constants.Engine.ThrustCoefficients
%   Throttle     - Throttle command input [-]
%   Sim_Extender - Scaling factor for simulation time [s]
%   pdynmc       - Dynamic pressure [Pa]
%   acowl        - Engine cowl area scaling factor [-]
%   IC           - Struct with constants (requires IC.AGRAV = gravity [m/s^2])
%   refa         - Reference area [m^2]
%
% OUTPUTS:
%   Thrust       - Propulsive thrust force [N]
%   fmdot        - Fuel mass depletion rate [kg/s]
%   cx_prop      - Propulsive force coefficient [-]
%
% METHOD:
%   1. Constrain throttle input to physical limits.
%   2. Interpolate Specific Impulse (SPI) and capture area from engine
%      coefficient tables as functions of Mach, throttle, and angle of attack.
%   3. Compute thrust using interpolated SPI, capture area, atmospheric
%      properties, and throttle input.
%   4. Compute the fuel mass depletion rate from thrust and SPI.
%   5. Compute the dimensionless propulsive force coefficient for coupling
%      with aerodynamic forces and moments.
%
% -------------------------------------------------------------------------

    % Constants
    thrtl_idle = 0.05;   % Minimum throttle setting
    thrtl_max  = 2;      % Maximum throttle setting
    AGRAV = Sim.earth.AGRAV;    % Gravitational acceleration [m/s^2]
    acowl = Sim.vehicle.acowl;

    % Breakpoints from engine coefficient tables
    Mach_vec     = Data.ThrustCoefficients.Mach_vec;
    alpha_vec    = Data.ThrustCoefficients.alpha_vec;
    throttle_vec = Data.ThrustCoefficients.throttle_vec;

    % Tables for thrust modeling
    capture_area_tab = Data.ThrustCoefficients.Capture_A;
    SPI_tab          = Data.ThrustCoefficients.SPI_tab;

    % Apply throttle limits
    Throttle = max(min(Throttle, thrtl_max), thrtl_idle);

    % Interpolate Specific Impulse (SPI) from Mach-throttle table
    SPI = interp2(Mach_vec, throttle_vec, SPI_tab, Mach, Throttle, 'linear');

    % Interpolate capture area from Mach-alpha table
    capture_area = interp2(Mach_vec, alpha_vec, capture_area_tab, Mach, alphax, 'linear');

    % Compute thrust [N]
    Thrust = SPI * 0.029 * Throttle * AGRAV * rho * DVBA * capture_area * acowl;

end

== matlab function Trim/Airframe/Environment/ENVIRONMENT/Magnitude ==
  data: VBAD input; dvba output
function dvba = fcn(VBAD)

dvba = sqrt(VBAD(1)^2+VBAD(2)^2+VBAD(3)^2);

== matlab function Trim/Airframe/Newton and Euler/NEWTON/Geodetic Position Update/Find Geodetic Position ==
  data: SBII input; lon output; Sim parameter; lat output; alt output
function [lon, lat, alt] = cad_geo84_in_cont(SBII, Sim)

    FLATTENING  = Sim.earth.FLATTENING;
    SMAJOR_AXIS = Sim.earth.SMAJOR_AXIS;
    GW_CLONG    = Sim.earth.GW_CLONG;
    % Earth's eccentricity squared

    e2 = 2 * FLATTENING - FLATTENING^2;
    % Extract position
    x = SBII(1);
    y = SBII(2);
    z = SBII(3);

    % Compute longitude first
    lon_inertial = atan2(y, x);
    lon = lon_inertial  - GW_CLONG;

    % Normalize longitude to (-pi, pi)
    lon = atan2(sin(lon), cos(lon));

    % Compute preliminary values
    rho = sqrt(x^2 + y^2);
    dbi = sqrt(x^2 + y^2 + z^2);

    % Compute geocentric latitude
    lat_gc = atan2(z, rho);

    % Compute geodetic latitude using simple approximation
    lat = atan2(z + e2 * SMAJOR_AXIS * sin(lat_gc)^3, rho - e2 * SMAJOR_AXIS * cos(lat_gc)^3);

    % Radius of curvature in prime vertical
    N = SMAJOR_AXIS / sqrt(1 - e2 * sin(lat)^2);

    % Altitude
    alt = rho / cos(lat_gc) - N;
end

== matlab function Trim/Airframe/Newton and Euler/NEWTON/Geodetic Position Update/Inertial to Geodetic ==
  data: lon input; TDI output; lat output; lon output; lat input; alt input; Sim parameter; alt output
function [TDI, lat, lon, alt] = cad_tdi84( lon, lat, alt, Sim)

%     GW_CLONG = Sim.earth.GW_CLONG;
% 
%     % Compute celestial longitude of the vehicle at simulation 'time'
%     lon_cel = GW_CLONG + lon;
% 
%     % Compute transformation matrix elements
%     tdi13 = cos(lat);
%     tdi33 = -sin(lat);
%     tdi22 = cos(lon_cel);
%     tdi21 = -sin(lon_cel);
% 
%     % Construct the transformation matrix
%     TDI = [ tdi33 * tdi22, -tdi33 * tdi21, tdi13;
%             tdi21,         tdi22,          0;
%            -tdi13 * tdi22,  tdi13 * tdi21, tdi33 ];
     TDI =   [   0     0     1;
      0     1     0;
     -1     0     0];
end

== matlab function Trim/Airframe/Environment/ENVIRONMENT/Atmosphere calculation ==
  data: rho output; press output; tempk output; vsound output; alt_km input
function [rho, press, tempk,vsound] = us76_nasa2002(alt_km)
    % 1976 US Standard Atmosphere Model
    % Inputs:
    %   z  - Altitude (km)
    % Outputs:
    %   d  - Density (kg/m^3)
    %   p  - Pressure (Pa)
    %   t  - Temperature (K)
    %   s  - Speed of sound (m/s)
    %   status - Returns 0 if altitude is in range, 1 if out of range

    % Initialize all outputs to avoid "not fully defined" errors
  
    rho = 0;
    press = 0;
    tempk = 0;
    vsound = 0;

    % Constants
    ro = 6356.766;  % Earth radius (km)
    go = 9.80665;   % Gravity (m/s^2)
    wmo = 28.9644;  % Molecular weight (dimensionless)
    rs = 8314.32;   % Universal gas constant (J/kmol-K)

    % Altitude table (km)
    zs = [0, 11.019, 20.063, 32.162, 47.35, 51.413, 71.802, 86, 91, 94, ...
          97, 100, 103, 106, 108, 110, 112, 115, 120, 125, 130, 135, 140, ...
          145, 150, 155, 160, 165, 170, 180, 190, 210, 230, 265, 300, 350, ...
          400, 450, 500, 550, 600, 650, 700, 750, 800, 850, 900, 950, 1000];

    % Temperature table (K)
    tms = [288.15, 216.65, 216.65, 228.65, 270.65, 270.65, 214.65, ...
           186.95, 186.87, 187.74, 190.40, 195.08, 202.23, 212.89, ...
           223.29, 240.00, 264.00, 300.00, 360.00, 417.23, 469.27, ...
           516.59, 559.63, 598.78, 634.39, 666.80, 696.29, 723.13, ...
           747.57, 790.07, 825.31, 878.84, 915.78, 955.20, 976.01, ...
           990.06, 995.83, 998.22, 999.24, 999.67, 999.85, 999.93, ...
           999.97, 999.99, 999.99, 1000, 1000, 1000, 1000];

    % Molecular weight table
    wms = [28.9644, 28.9644, 28.9644, 28.9644, 28.9644, 28.9644, ...
           28.9644, 28.9522, 28.8890, 28.7830, 28.6200, 28.3950, ...
           28.1040, 27.7650, 27.5210, 27.2680, 27.0200, 26.6800, ...
           26.2050, 25.8030, 25.4360, 25.0870, 24.7490, 24.4220, ...
           24.1030, 23.7920, 23.4880, 23.1920, 22.9020, 22.3420, ...
           21.8090, 20.8250, 19.9520, 18.6880, 17.7260, 16.7350, ...
           15.9840, 15.2470, 14.3300, 13.0920, 11.5050, 9.7180, ...
           7.9980, 6.5790, 5.5430, 4.8490, 4.4040, 4.1220, 3.9400];

    % Pressure table (hPa converted to Pa)
    ps = [1013.25, 226.32, 54.7487, 8.68014, 1.10905, 0.66938, ...
          0.039564, 3.7338e-03, 1.5381e-03, 9.0560e-04, 5.3571e-04, ...
          3.2011e-04, 1.9742e-04, 1.2454e-04, 9.3188e-05, 7.1042e-05, ...
          5.5547e-05, 4.0096e-05, 2.5382e-05, 1.7354e-05, 1.2505e-05, ...
          9.3568e-06, 7.2028e-06, 5.6691e-06, 4.5422e-06, 3.6930e-06, ...
          3.0395e-06, 2.5278e-06, 2.1210e-06, 1.5271e-06, 1.1266e-06, ...
          6.4756e-07, 3.9276e-07, 1.7874e-07, 8.7704e-08, 3.4498e-08, ...
          1.4518e-08, 6.4468e-09, 3.0236e-09, 1.5137e-09, 8.2130e-10, ...
          4.8865e-10, 3.1908e-10, 2.2599e-10, 1.7036e-10, 1.3415e-10, ...
          1.0873e-10, 8.9816e-11, 7.5138e-11] * 100;

    % Check altitude range
    if alt_km < 0 || alt_km > 1000
        rho = 0; press = 0; tempk = 0; vsound = 0;
        return;
    end

    % Find altitude index using bisection search
    i = 0;
    upper = length(zs) - 1;
    while (upper - i > 1)
        test = floor((i + upper) / 2);
        if alt_km > zs(test)
            i = test;
        else
            upper = test;
        end
    end

    if i < 7
        zl = ro * zs(i) / (ro + zs(i));
        zu = ro * zs(i+1) / (ro + zs(i+1));
        wm = wmo;
        ht = ro * alt_km / (ro + alt_km);
        g = (tms(i+1) - tms(i)) / (zu - zl);

        if g ~= 0
            press = ps(i) * (tms(i) / (tms(i) + g * (ht - zl)))^((go * wmo) / (rs * g * 0.001));
        else
            press = ps(i) * exp(-(go * wmo * (ht * 1000 - zl * 1000)) / (rs * tms(i)));
        end
        tempk = tms(i) + g * (ht - zl);
    else
        % Non-tropospheric layers
        if i == 7
            tempk = tms(8);
        elseif i >= 8 && i < 15
            tempk = 263.1905 - 76.3232 * sqrt(1 - ((alt_km - 91) / 19.9429)^2);
        elseif i >= 15 && i < 18
            tempk = 240 + 12 * (alt_km - 110);
        elseif i >= 18
            xi = (alt_km - 120) * (ro + 120) / (ro + alt_km);
            tempk = 1000 - 640 * exp(-0.01875 * xi);
        end

        % Interpolating pressure and molecular weight
        j = i;
        if i == 47, j = i - 1; end

        z0 = zs(j);
        z1 = zs(j+1);
        z2 = zs(j+2);

        wma = wms(j) * (alt_km - z1) * (alt_km - z2) / ((z0 - z1) * (z0 - z2)) + ...
              wms(j+1) * (alt_km - z0) * (alt_km - z2) / ((z1 - z0) * (z1 - z2)) + ...
              wms(j+2) * (alt_km - z0) * (alt_km - z1) / ((z2 - z0) * (z2 - z1));

        alpa = log(ps(j)) * (alt_km - z1) * (alt_km - z2) / ((z0 - z1) * (z0 - z2)) + ...
               log(ps(j+1)) * (alt_km - z0) * (alt_km - z2) / ((z1 - z0) * (z1 - z2)) + ...
               log(ps(j+2)) * (alt_km - z0) * (alt_km - z1) / ((z2 - z0) * (z2 - z1));

        alpb = alpa;
        wmb = wma;

        if i ~= 7 && i ~= 47
            j = j - 1;
            z0 = zs(j);
            z1 = zs(j+1);
            z2 = zs(j+2);
            alpb = log(ps(j)) * (alt_km - z1) * (alt_km - z2) / ((z0 - z1) * (z0 - z2)) + ...
                   log(ps(j+1)) * (alt_km - z0) * (alt_km - z2) / ((z1 - z0) * (z1 - z2)) + ...
                   log(ps(j+2)) * (alt_km - z0) * (alt_km - z1) / ((z2 - z0) * (z2 - z1));

            wmb = wms(j) * (alt_km - z1) * (alt_km - z2) / ((z0 - z1) * (z0 - z2)) + ...
                  wms(j+1) * (alt_km - z0) * (alt_km - z2) / ((z1 - z0) * (z1 - z2)) + ...
                  wms(j+2) * (alt_km - z0) * (alt_km - z1) / ((z2 - z0) * (z2 - z1));
        end

        press = 100 * exp((alpa + alpb) / 2);
        wm = (wma + wmb) / 2;
    end

    % Compute density and speed of sound
    rho = (wm * press) / (rs * tempk);
    vsound = sqrt(1.4 * press / rho);
end
